simulink model "untitled1"  (R2017a)
settings: Solver=VariableStepAuto  StartTime=0.0  StopTime=2  RelTol=1e-3
values from neighbouring files (symbols this model uses):
  As = [0  1  0; 0  0  1; 0  0  0]    [first.mat]
  Bs = [0 0 1]    [first.mat]
  Cs = [1 0 -0.042]    [first.mat]
libraries: simulink x1
settings Model: Creator=Shashi  LastModifiedBy=Shashi

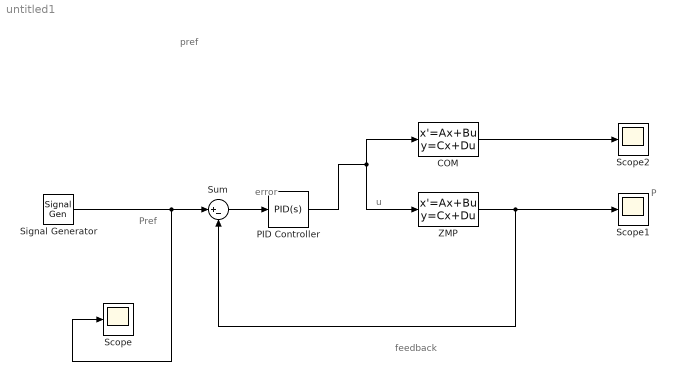
== system untitled1 ==
  note: error
  note: u
  note: P
  note: Pref
  note: feedback
  note: pref
  COM : StateSpace  A=As  B=Bs  C=Cs  D=0  X0=0  ContinuousStateAttributes='parameter'
  PID Controller : simulink/Continuous/PID Controller  Controller=PID  TimeDomain=Continuous-time  SampleTime=-1  IntegratorMethod=Forward Euler  FilterMethod=Forward Euler  Form=Parallel  UseFilter=on  ControllerParametersSource=internal  P=-123719.154595778  I=-119049954.533653  D=-4.31281198664873  N=19867.4502555126  InitialConditionSource=internal  InitialConditionForIntegrator=0  InitialConditionForFilter=0  ExternalReset=none  LimitOutput=off  UpperSaturationLimit=inf  LowerSaturationLimit=-inf  LinearizeAsGain=on  AntiWindupMode=none  Kb=1  TrackingMode=off  Kt=1  PParamMin=[]  PParamMax=[]  IParamMin=[]  IParamMax=[]  DParamMin=[]  DParamMax=[]  NParamMin=[]  NParamMax=[]  KbParamMin=[]  KbParamMax=[]  KtParamMin=[]  KtParamMax=[]  POutMin=[]  POutMax=[]  IOutMin=[]  IOutMax=[]  DOutMin=[]  DOutMax=[]  NOutMin=[]  NOutMax=[]  KbOutMin=[]  KbOutMax=[]  KtOutMin=[]  KtOutMax=[]  IntegratorOutMin=[]  IntegratorOutMax=[]  FilterOutMin=[]  FilterOutMax=[]  SumOutMin=[]  SumOutMax=[]  SumI1OutMin=[]  SumI1OutMax=[]  SumI2OutMin=[]  SumI2OutMax=[]  SumI3OutMin=[]  SumI3OutMax=[]  SumDOutMin=[]  SumDOutMax=[]  SaturationOutMin=[]  SaturationOutMax=[]  IntegratorContinuousStateAttributes=''  IntegratorStateMustResolveToSignalObject=off  IntegratorRTWStateStorageClass=Auto  FilterContinuousStateAttributes=''  FilterStateMustResolveToSignalObject=off  FilterRTWStateStorageClass=Auto  DifferentiatorICPrevScaledInput=0  DifferentiatorOutMin=[]  DifferentiatorOutMax=[]  InitialConditionSetting=State (most efficient)
  Scope : Scope
  Scope1 : Scope
  Scope2 : Scope
  Signal Generator : SignalGenerator  WaveForm=square  Amplitude=3  Frequency=0.5
  Sum : Sum  Inputs=|+-
  ZMP : StateSpace  A=As  B=Bs  C=Cs  D=0  X0=0  ContinuousStateAttributes='parameter'
  wires:
  Signal Generator/1 -> Sum/1, Scope/1
  Sum/1 -> PID Controller/1
  ZMP/1 -> Scope1/1, Sum/2
  COM/1 -> Scope2/1
  PID Controller/1 -> COM/1, ZMP/1
